simulink model "sil_test"  (R2022b)
settings: Solver=VariableStepAuto  StartTime=0.0  StopTime=inf  RelTol=1e-3
undefined symbols (not defined in the file): battery_monitor, battery_monitor_lib, BM_STATUSES, canChannel, DI_STATUSES, driver_interface, driver_interface_lib, Ended, governor, governor_lib, MI_STATUSES, motor_interface, motor_interface_lib, simp_vd_interface, simp_vd_lib, Single
libraries: canmsglib x16, canlib x10, simulink x6, speedgoatlib_IO191 x5, slrealtimeiplib x3, AMK_comms_plant_lib x1, BMS_plant_lib x1, speedgoatlib_IO614 x1, slrealtimeutilitieslib x1, etargetslib x1
(part 1 of 3)
settings Model: Creator=maxfa  LastModifiedBy=maxfa

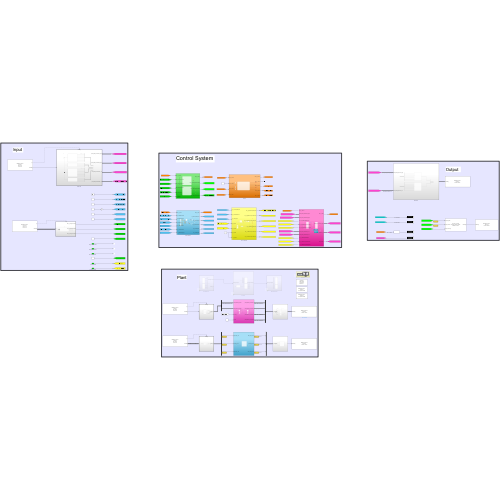
[thumbnail: Simulink's stored preview of the top-level diagram]
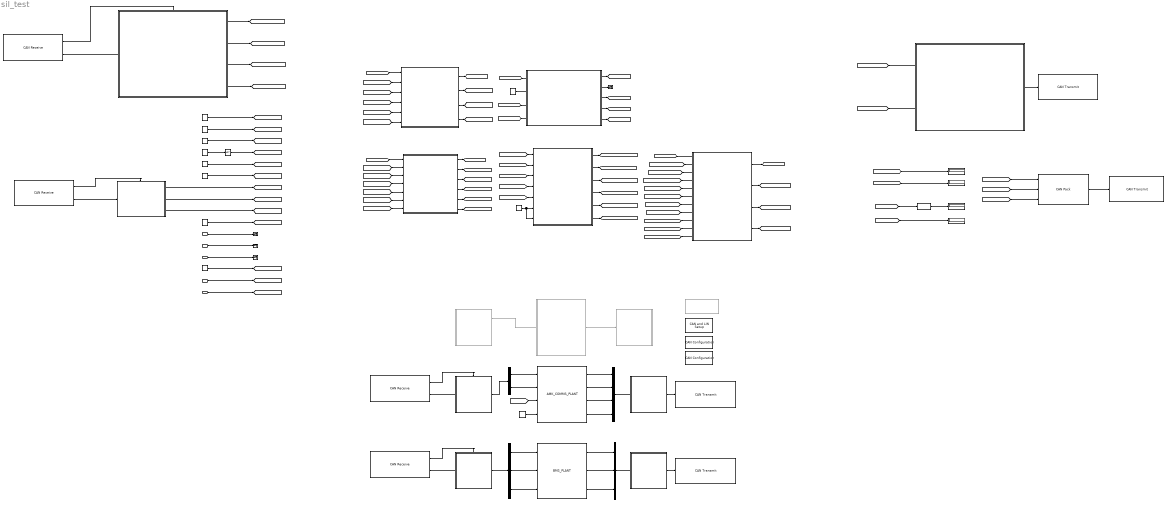
== system sil_test ==
  note: Plant
  note: Control System
  note: Input
  note: Output
  BM_LowThermValue : Inport  OutDataTypeStr=int8  Unit=°C
  BM_HighThermValue : Inport  Port=2  OutDataTypeStr=int8  Unit=°C
  BM_AvgThermValue : Inport  Port=3  OutDataTypeStr=int8  Unit=°C
  VD_LFWheelSpeed : Inport  Port=4  OutDataTypeStr=int16  Unit=rpm
  VD_RFWheelSpeed : Inport  Port=5  OutDataTypeStr=int16  Unit=rpm
  AMK_COMMS_PLANT : AMK_comms_plant_lib/AMK_COMMS_PLANT  SystemSampleTime=-1  VariantActivationTime=update diagram  Latency=0  AutoFrameSizeCalculation=off
  AMK_Input : Subsystem  TreatAsAtomicUnit=on
  AMK_Output : Subsystem
  BMS_PLANT : BMS_plant_lib/BMS_PLANT  SystemSampleTime=-1  VariantActivationTime=update diagram  Latency=0  AutoFrameSizeCalculation=off
  Bus Creator : BusCreator  Inputs=4
  Bus Creator1 : BusCreator  Inputs=3
  Bus Selector : BusSelector  OutputSignals=ptCAN_AMK0_Setpoints1_Left,ptCAN_AMK1_Setpoints1_Right
  Bus Selector1 : BusSelector  OutputSignals=AIR_pos,precharge,AIR_neg
  CAN Configuration : canlib/CAN Configuration  BlockHandle=2172.0005  Device=MathWorks Virtual 1 (Channel 1)  DeviceMenu=MathWorks Virtual 1 (Channel 1)  ObjConstructor=canChannel('MathWorks', 'Virtual 1', 1)  BusSpeed=500000  EnableBitParameters=off  AckMode=Normal
  CAN Configuration1 : canlib/CAN Configuration  BlockHandle=2172.0005  Device=MathWorks Virtual 1 (Channel 2)  DeviceMenu=MathWorks Virtual 1 (Channel 2)  ObjConstructor=canChannel('MathWorks', 'Virtual 1', 2)  BusSpeed=500000  EnableBitParameters=off  AckMode=Normal
  CAN Pack : canmsglib/CAN Pack  CANdbFile=C:\Users\maxfa\Documents\vehicle_control_system\src\testing\Vehicle_HIL_plant\VEH_CAN.dbc  MsgList=Contactor_States  MsgName=Contactor_States  MsgIDType=Standard (11-bit identifier)  MsgIdentifier=1570  MsgLength=3  Remote=off  ApplyMinMax=off  BusOutput=off  SignalInfo={'Pack_Negative','16','8','LE','unsigned','Standard','0','1','0','-Inf','Inf';'Pack_Positive','0','8','LE','unsigned','Standard','0','1','0','-Inf','Inf';'Pack_Precharge','8','8','LE','unsigned','Standard','0','1','0','-Inf','Inf'}
      settings: LibrarySourceBlock=canlib/CAN Pack  DataFormat=CANdb specified signals
  CAN Receive : canlib/CAN Receive  BlockHandle=204.0002  Device=MathWorks Virtual 1 (Channel 1)  DeviceMenu=MathWorks Virtual 1 (Channel 1)  ObjConstructor=canChannel('MathWorks', 'Virtual 1', 1)  EnableStandardIDsFilter=off  StdIDsCombo=Allow all  StandardIDs=0  EnableExtendedIDsFilter=off  ExtIDsCombo=Allow all  ExtendedIDs=0  SampleTime=0.005  MsgsPerTimestep=all  InternalFilterUpdateStatus=on  BusOutput=off
  CAN Receive1 : canlib/CAN Receive  BlockHandle=207.0002  Device=MathWorks Virtual 1 (Channel 1)  DeviceMenu=MathWorks Virtual 1 (Channel 1)  ObjConstructor=canChannel('MathWorks', 'Virtual 1', 1)  EnableStandardIDsFilter=off  StdIDsCombo=Allow all  StandardIDs=0  EnableExtendedIDsFilter=off  ExtIDsCombo=Allow all  ExtendedIDs=0  SampleTime=0.005  MsgsPerTimestep=all  InternalFilterUpdateStatus=on  BusOutput=off
  CAN Receive2 : canlib/CAN Receive  BlockHandle=210.0002  Device=MathWorks Virtual 1 (Channel 2)  DeviceMenu=MathWorks Virtual 1 (Channel 2)  ObjConstructor=canChannel('MathWorks', 'Virtual 1', 2)  EnableStandardIDsFilter=off  StdIDsCombo=Allow all  StandardIDs=0  EnableExtendedIDsFilter=off  ExtIDsCombo=Allow all  ExtendedIDs=0  SampleTime=0.005  MsgsPerTimestep=all  InternalFilterUpdateStatus=on  BusOutput=on
  CAN Receive4 : canlib/CAN Receive  BlockHandle=213.0002  Device=MathWorks Virtual 1 (Channel 2)  DeviceMenu=MathWorks Virtual 1 (Channel 2)  ObjConstructor=canChannel('MathWorks', 'Virtual 1', 2)  EnableStandardIDsFilter=off  StdIDsCombo=Allow all  StandardIDs=0  EnableExtendedIDsFilter=off  ExtIDsCombo=Allow all  ExtendedIDs=0  SampleTime=0.005  MsgsPerTimestep=all  InternalFilterUpdateStatus=on  BusOutput=on
  CAN Transmit : canlib/CAN Transmit  BlockHandle=216.0002  Device=MathWorks Virtual 1 (Channel 1)  DeviceMenu=MathWorks Virtual 1 (Channel 1)  ObjConstructor=canChannel('MathWorks', 'Virtual 1', 1)  EnableEventTransmit=off  EnablePeriodicTransmit=on  MessagePeriod=0.005
  CAN Transmit1 : canlib/CAN Transmit  BlockHandle=218.0002  Device=MathWorks Virtual 1 (Channel 1)  DeviceMenu=MathWorks Virtual 1 (Channel 1)  ObjConstructor=canChannel('MathWorks', 'Virtual 1', 1)  EnableEventTransmit=off  EnablePeriodicTransmit=on  MessagePeriod=0.005
  CAN Transmit2 : canlib/CAN Transmit  BlockHandle=3044.0012  Device=MathWorks Virtual 1 (Channel 2)  DeviceMenu=MathWorks Virtual 1 (Channel 2)  ObjConstructor=canChannel('MathWorks', 'Virtual 1', 2)  EnableEventTransmit=off  EnablePeriodicTransmit=on  MessagePeriod=0.005
  CAN Transmit4 : canlib/CAN Transmit  BlockHandle=220.0002  Device=MathWorks Virtual 1 (Channel 2)  DeviceMenu=MathWorks Virtual 1 (Channel 2)  ObjConstructor=canChannel('MathWorks', 'Virtual 1', 2)  EnableEventTransmit=off  EnablePeriodicTransmit=on  MessagePeriod=0.005
  "CAN and LIN Setup " : speedgoatlib_IO614/CAN and LIN Setup   moduleInitValues="[614    1    1   -1   -1]"  id=1  moduleType=IO614  pciSlot=-1  canChn1=CAN (HS)  canChn2=CAN (HS)  canChn3=Disabled  canChn4=Disabled  linChn1=Disabled  linChn2=Disabled  canInitStructArray=[]  canTermStructArray=[]  canChn1InitValues="[2   4   1  31   8   2   1   5   2]"  arbBdrChn1=500 kBaud  arbManBdrChn1=[4,1,31,8]  fdBdrChn1=5.0 MBaud  fdManBdrChn1=[2,1,5,2]  canChn2InitValues="[2   4   1  31   8   2   1   5   2]"  arbBdrChn2=500 kBaud  arbManBdrChn2=[4,1,31,8]  fdBdrChn2=5.0 MBaud  fdManBdrChn2=[2,1,5,2]  canChn3InitValues="[1   2   1  31   8   2   1   5   2]"  arbBdrChn3=1.0 MBaud  arbManBdrChn3=[2,1,31,8]  fdBdrChn3=5.0 MBaud  fdManBdrChn3=[2,1,5,2]  canChn4InitValues="[1   2   1  31   8   2   1   5   2]"  arbBdrChn4=1.0 MBaud  arbManBdrChn4=[2,1,31,8]  fdBdrChn4=5.0 MBaud  fdManBdrChn4=[2,1,5,2]  bdrLIN1=19200  linChn1InitValues="[1  19200]"  bdrLIN2=19200  linChn2InitValues="[1  19200]"
      settings: LibrarySourceBlock=speedgoatlib_CANLIN_OfA2/CAN and LIN Setup
  Cast To Single : DataTypeConversion  OutDataTypeStr=uint8  SaturateOnIntegerOverflow=off  RndMeth=Floor
  Constant : Constant  Value=0
  Constant1 : Constant  Value=0
  Constant13 : Constant  Value=0  OutMin=0  OutMax=1
  Constant14 : Constant  Value=100  OutMin=0  OutMax=100
  Constant2 : Constant  Value=0
  Constant4 : Constant  Value=0.5066380718954249  OutMin=0  OutMax=1
  Constant5 : Constant  OutMin=0  OutMax=1
  Constant6 : Constant  OutMin=0  OutMax=1
  Constant7 : Constant  Value=0  OutMin=0  OutMax=1
  Constant8 : Constant  Value=0  OutMin=0  OutMax=1
  Constant9 : Constant  Value=0.02343014359698682  OutMin=0  OutMax=1
  Dashboard : Subsystem  Commented=on
  Display{,1..3} (4 alike) : Display
  Function-Call Subsystem : Subsystem  TreatAsAtomicUnit=on
  Function-Call Subsystem1 : Subsystem  TreatAsAtomicUnit=on
  Function-Call Subsystem2 : Subsystem  TreatAsAtomicUnit=on
  NOT : Logic  Operator=NOT  IconShape=distinctive  AllPortsSameDT=off  OutDataTypeStr=boolean
  Speedgoat Inputs : Subsystem  Commented=on
  Speedgoat Outputs : Subsystem  Commented=on
  Subsystem : Subsystem
  Subsystem1 : Subsystem
  TCP Server : Subsystem  Commented=on
  Terminator{,1..3} (4 alike) : Terminator
  battery_monitor : Subsystem  AncestorBlock=battery_monitor_lib/battery_monitor
  driver_interface : Subsystem  AncestorBlock=driver_interface_lib/driver_interface
  governor : Subsystem  AncestorBlock=governor_lib/governor
  motor_interface : Subsystem  AncestorBlock=motor_interface_lib/motor_interface
  simp_vd_interface : Subsystem  AncestorBlock=simp_vd_lib/simp_vd_interface
  wires:
  Function-Call Subsystem1/1(pt_CAN_IN) -> Bus Selector1/1
  Bus Selector1/2 -> BMS_PLANT/2  "<precharge>"
  BMS_PLANT/3 -> Bus Creator1/3  "AIR_neg_sts"
  Subsystem1/1(Out1) -> CAN Transmit4/1
  Bus Selector1/1 -> BMS_PLANT/1  "<AIR_pos>"
  AMK_COMMS_PLANT/4 -> Bus Creator/4  "ptCAN_AMK1_ActualValues2"
  CAN Receive2/2 -> Function-Call Subsystem1/1(In1)
  BMS_PLANT/2 -> Bus Creator1/2  "precharge_sts"
  AMK_COMMS_PLANT/3 -> Bus Creator/3  "ptCAN_AMK1_ActualValues1"
  Subsystem/1(Out1) -> CAN Transmit1/1
  TCP Server/1(Speedgoat Outputs) -> Speedgoat Outputs/1(Speedgoat Outputs)
  AMK_COMMS_PLANT/2 -> Bus Creator/2  "ptCAN_AMK0_ActualValues2"
  Bus Creator1/1 -> Subsystem1/1(pt_CAN_OUT)
  CAN Receive1/2 -> Function-Call Subsystem/1(In1)
  Function-Call Subsystem/1(pt_CAN_IN) -> Bus Selector/1
  Constant/1 -> AMK_COMMS_PLANT/4
  Bus Selector1/3 -> BMS_PLANT/3  "<AIR_neg>"
  BMS_PLANT/1 -> Bus Creator1/1  "AIR_pos_sts"
  Bus Creator/1 -> Subsystem/1(pt_CAN_OUT)
  Bus Selector/2 -> AMK_COMMS_PLANT/2  "<ptCAN_AMK1_Setpoints1_Right>"
  AMK_COMMS_PLANT/1 -> Bus Creator/1  "ptCAN_AMK0_ActualValues1"
  Bus Selector/1 -> AMK_COMMS_PLANT/1  "<ptCAN_AMK0_Setpoints1_Left>"
  Speedgoat Inputs/1(Speedgoat Inputs) -> TCP Server/1(Speedgoat Inputs)
  [BM_b_prechargeContactorCMD] -> CAN Pack/3
  BM_AvgThermValue/1 -> Terminator3/1
  motor_interface/2(ptCAN_AMK_Setpoints1_Right) -> [ptCAN_AMK_Setpoints1_Right]
  Constant14/1 -> [BM_PackSOC]
  BM_HighThermValue/1 -> Terminator2/1
  [BM_PackSOC] -> battery_monitor/6(BM_PackSOC)
  VD_LFWheelSpeed/1 -> [VD_LFWheelSpeed]
  Constant6/1 -> [DI_RearBrakePressure]
  [BM_HVnegContactorSts] -> battery_monitor/4(BM_HVnegContactorSts)
  [VD_RFWheelSpeed] -> simp_vd_interface/5(DI_p_wspdRF)
  battery_monitor/4(BM_b_HVnegContactorCMD) -> [BM_b_HVnegContactorCMD]
  [VD_LFWheelSpeed] -> simp_vd_interface/4(DI_p_wspdLF)
  VD_RFWheelSpeed/1 -> [VD_RFWheelSpeed]
  Constant4/1 -> [DI_SteeringAngle]
  [DI_StartButton] -> driver_interface/4(DI_StartButton)
  motor_interface/1(GOV_e_miSts) -> [GOV_e_miSts]
  BM_LowThermValue/1 -> Terminator1/1
  [GOV_e_miCmd] -> motor_interface/1(GOV_e_miCmd)
  [BM_HvilFeedback] -> battery_monitor/5(BM_HvilFeedback)
  [DI_AccelPedalPosition2] -> driver_interface/6(DI_V_AccelPedalPos2)
  [DI_b_brakeLightEn] -> Display1/1  "DI_b_brakeLightEn"
  [GOV_e_diSts] -> governor/4(GOV_e_diSts)
  Cast To Single/1 -> Display2/1
  [DI_p_brakePedalPosition] -> simp_vd_interface/2(DI_p_brakePedalPosition)
  [GOV_e_govSts] -> Cast To Single/1  "GOV_e_govSts"
  [MI_InverterEn] -> Display3/1
  simp_vd_interface/1(VD_n_RightMotorSpeedRequest) -> [VD_n_RightMotorSpeedRequest]
  governor/4(GOV_e_diCmd) -> [GOV_e_diCmd]
  [DI_RearBrakePressure] -> driver_interface/3(DI_RearBrakePressure)
  motor_interface/4(MI_InverterEn) -> [MI_InverterEn]
  battery_monitor/2(BM_b_prechargeContactorCMD) -> [BM_b_prechargeContactorCMD]
  [GOV_e_diCmd] -> driver_interface/1(GOV_e_diCmd)
  [DI_AccelPedalPosition1] -> driver_interface/5(DI_V_AccelPedalPos1)
  [ptCAN_AMK_ActualValues2_Left] -> motor_interface/8(ptCAN_AMK_ActualValues2_Left)
  [DI_SteeringAngle] -> driver_interface/7(Dl_V_RawSteeringAngle)
  simp_vd_interface/3(VD_T_RightMotorTorqueLimitNegative) -> [VD_T_RightMotorTorqueLimitNegative]
  [DI_FrontBrakePressure] -> driver_interface/2(DI_FrontBrakePressure)
  governor/5(GOV_e_govSts) -> [GOV_e_govSts]
  [BM_prechrgContactorSts] -> battery_monitor/2(BM_prechrgContactorSts)
  driver_interface/6(DI_b_brakeLightEn) -> [DI_b_brakeLightEn]
  simp_vd_interface/6(VD_T_LeftMotorTorqueLimitNegative) -> [VD_T_LeftMotorTorqueLimitNegative]
  simp_vd_interface/5(VD_T_LeftMotorTorqueLimitPositive) -> [VD_T_LeftMotorTorqueLimitPositive]
  [ptCAN_AMK_ActualValues1_Left] -> motor_interface/7(ptCAN_AMK_ActualValues1_Left)
  simp_vd_interface/2(VD_T_RightMotorTorqueLimitPositive) -> [VD_T_RightMotorTorqueLimitPositive]
  Constant13/1 -> [BM_HvilFeedback]
  [DI_p_driverTorqueRequest] -> simp_vd_interface/1(DI_p_driverTorqueRequest)
  [GOV_e_bmCmd] -> battery_monitor/1(GOV_e_bmCmd)
  simp_vd_interface/4(VD_n_LeftMotorSpeedRequest) -> [VD_n_LeftMotorSpeedRequest]
  Constant5/1 -> [DI_FrontBrakePressure]
  [VD_T_LeftMotorTorqueLimitPositive] -> motor_interface/10(VD_T_LeftMotorTorqueLimitPositive)
  [ptCAN_AMK_ActualValues2_Right] -> motor_interface/3(ptCAN_AMK_ActualValues2_Right)
  Function-Call Subsystem2/1(BM_b_prechrgContactorSts) -> [BM_prechrgContactorSts]
  governor/1(GOV_e_bmCmd) -> [GOV_e_bmCmd]
  [GOV_e_miSts] -> governor/3(GOV_e_miSts)
  governor/3(GOV_e_miCmd) -> [GOV_e_miCmd]
  Function-Call Subsystem2/3(BM_b_HVnegContactorSts) -> [BM_HVnegContactorSts]
  Constant9/1 -> [DI_AccelPedalPosition2]
  [BM_HVposContactorSts] -> battery_monitor/3(BM_HVposContactorSts)
  [VD_n_RightMotorSpeedRequest] -> motor_interface/4(VD_n_RightMotorSpeedRequest)
  [VD_T_RightMotorTorqueLimitNegative] -> motor_interface/6(VD_T_RightMotorTorqueLimitNegative)
  driver_interface/2(DI_driverTorqueRequest) -> [DI_p_driverTorqueRequest]
  Constant7/1 -> NOT/1
  Constant1/1 -> governor/2(GOV_e_vdSts)
  driver_interface/1(GOV_e_diSts) -> [GOV_e_diSts]
  [GOV_e_bmSts] -> governor/1(GOV_e_bmSts)
  [VD_T_RightMotorTorqueLimitPositive] -> motor_interface/5(VD_T_RightMotorTorqueLimitPositive)
  Function-Call Subsystem2/2(BM_b_HVposContactorSts) -> [BM_HVposContactorSts]
  driver_interface/5(DI_b_driverSpeaker) -> [DI_b_driverSpeaker]
  driver_interface/3(DI_p_steeringAngle) -> [DI_p_steeringAngle]
  driver_interface/4(DI_p_brakePedalPos) -> [DI_p_brakePedalPosition]
  [ptCAN_AMK_ActualValues1_Right] -> motor_interface/2(ptCAN_AMK_ActualValues1_Right)
  [VD_T_LeftMotorTorqueLimitNegative] -> motor_interface/11(VD_T_LeftMotorTorqueLimitNegative)
  [DI_p_steeringAngle] -> simp_vd_interface/3(DI_p_steeringAngle)
  Constant8/1 -> [DI_AccelPedalPosition1]
  [DI_b_driverSpeaker] -> Display/1  "DI_b_driverSpeaker"
  governor/2(GOV_e_vdCmd) -> Terminator/1
  battery_monitor/1(GOV_e_bmSts) -> [GOV_e_bmSts]
  motor_interface/3(ptCAN_AMK_Setpoints1_Left) -> [ptCAN_AMK_Setpoints1_Left]
  [VD_n_LeftMotorSpeedRequest] -> motor_interface/9(VD_n_LeftMotorSpeedRequest)
  battery_monitor/3(BM_b_HVposContactorCMD) -> [BM_b_HVposContactorCMD]
  Constant2/1 -> simp_vd_interface/7(DI_p_wspdLRR), simp_vd_interface/6(DI_p_wspdLR)
  CAN Receive/1 -> AMK_Input/Trigger
  AMK_Input/4(ptCAN_AMK_ActualValues2_Left) -> [ptCAN_AMK_ActualValues2_Left]
  AMK_Input/2(ptCAN_AMK_ActualValues2_Right) -> [ptCAN_AMK_ActualValues2_Right]
  CAN Receive/2 -> AMK_Input/1(In1)
  AMK_Input/1(ptCAN_AMK_ActualValues1_Right) -> [ptCAN_AMK_ActualValues1_Right]
  AMK_Input/3(ptCAN_AMK_ActualValues1_Left) -> [ptCAN_AMK_ActualValues1_Left]
  CAN Receive4/2 -> Function-Call Subsystem2/1(In1)
  CAN Receive4/1 -> Function-Call Subsystem2/Trigger
  AMK_Output/1(Out1) -> CAN Transmit/1
  [ptCAN_AMK_Setpoints1_Right] -> AMK_Output/1(ptCAN_AMK_Setpoints1_Right)  "ptCAN_AMK_Setpoints1_Right"
  [ptCAN_AMK_Setpoints1_Left] -> AMK_Output/2(ptCAN_AMK_Setpoints1_Left)  "ptCAN_AMK_Setpoints1_Left"
  CAN Receive1/1 -> Function-Call Subsystem/Trigger
  CAN Receive2/1 -> Function-Call Subsystem1/Trigger
  [MI_InverterEn] -> AMK_COMMS_PLANT/3
  NOT/1 -> [DI_StartButton]
  CAN Pack/1 -> CAN Transmit2/1
  [BM_b_HVposContactorCMD] -> CAN Pack/2
  [BM_b_HVnegContactorCMD] -> CAN Pack/1

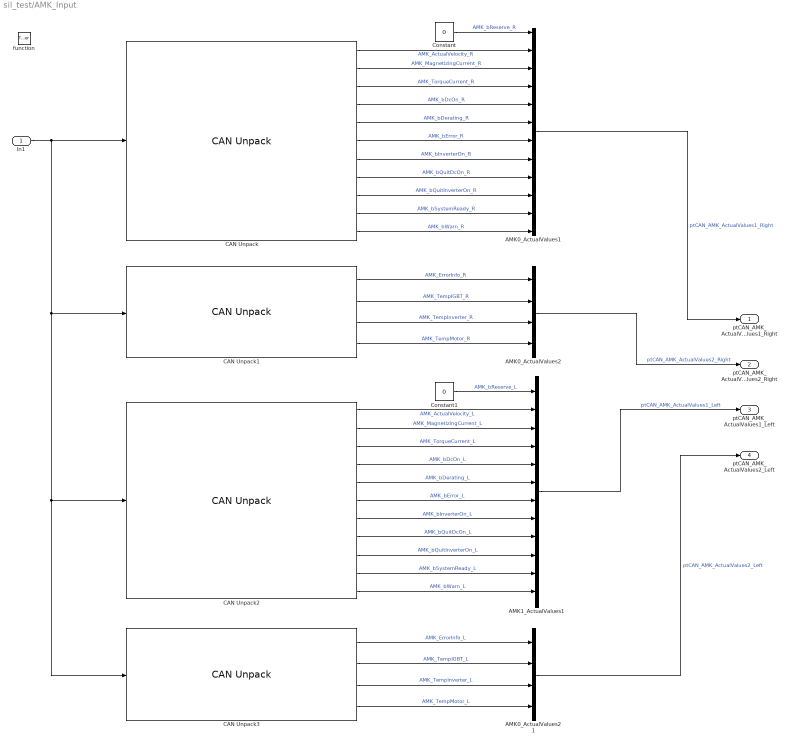
== system sil_test/AMK_Input ==
  In1 : Inport
  function : TriggerPort  TriggerType=function-call  VariantControl=(inherit)
  "AMK0_ActualValues1 " : BusCreator  Inputs=12
  "AMK0_ActualValues2 " : BusCreator  Inputs=4
  AMK0_ActualValues2 1 : BusCreator  Inputs=4
  AMK1_ActualValues1 : BusCreator  Inputs=12
  CAN Unpack : canmsglib/CAN Unpack  CANdbFile=C:\Users\maxfa\OneDrive\Documents\vehicle_control_system\src\testing\Plant\Bench\CAN_Databases-master\CAN_AMKInverter.dbc  MsgList=AMK1_ActualValues1  MsgName=AMK1_ActualValues1  MsgIDType=Standard (11-bit identifier)  MsgIdentifier=645  MsgLength=8  SignalInfo={'AMK_ActualVelocity','16','16','LE','signed','Standard','0','1','0','-Inf','Inf';'AMK_MagnetizingCurrent','48','16','LE','signed','Standard','0','1','0','-Inf','Inf';'AMK_TorqueCurrent','32','16','LE','signed','Standard','0','1','0','-Inf','Inf';'AMK_bDcOn','12','1','LE','unsigned','Standard','0','1','0','-Inf','Inf';'AMK_bDerating','15','1','LE','unsigned','Standard','0','1','0','-Inf','Inf';'AMK_bError','9','1','LE','unsigned','Standard','0','1','0','-Inf','Inf';'AMK_bInverterOn','14','1','LE','unsigned','Standard','0','1','0','-Inf','Inf';'AMK_bQuitDcOn','11','1','LE','unsigned','Standard','0','1','0','-Inf','Inf';'AMK_bQuitInverterOn','13','1','LE','unsigned','Standard','0','1','0','-Inf','Inf';'AMK_bSystemReady','8','1','LE','unsigned','Standard','0','1','0','-Inf','Inf';'AMK_bWarn','10','1','LE','unsigned','Standard','0','1','0','-Inf','Inf'}  IDPort=off  TimestampPort=off  ErrorPort=off  RemotePort=off  LengthPort=off  StatusPort=off  ApplyMinMax=off
      settings: LibrarySourceBlock=canlib/CAN Unpack  DataFormat=CANdb specified signals
  CAN Unpack1 : canmsglib/CAN Unpack  CANdbFile=C:\Users\maxfa\OneDrive\Documents\vehicle_control_system\src\testing\Plant\Bench\CAN_Databases-master\CAN_AMKInverter.dbc  MsgList=AMK1_ActualValues2  MsgName=AMK1_ActualValues2  MsgIDType=Standard (11-bit identifier)  MsgIdentifier=647  MsgLength=8  SignalInfo={'AMK_ErrorInfo','32','16','LE','unsigned','Standard','0','1','0','0','65535';'AMK_TempIGBT','48','16','LE','signed','Standard','0','0.1','0','-3276.8','3276.7';'AMK_TempInverter','16','16','LE','signed','Standard','0','0.1','0','-3276.8','3276.7';'AMK_TempMotor','0','16','LE','signed','Standard','0','0.1','0','-3276.8','3276.7'}  IDPort=off  TimestampPort=off  ErrorPort=off  RemotePort=off  LengthPort=off  StatusPort=off  ApplyMinMax=off
      settings: LibrarySourceBlock=canlib/CAN Unpack  DataFormat=CANdb specified signals
  CAN Unpack2 : canmsglib/CAN Unpack  CANdbFile=C:\Users\maxfa\OneDrive\Documents\vehicle_control_system\src\testing\Plant\Bench\CAN_Databases-master\CAN_AMKInverter.dbc  MsgList=AMK0_ActualValues1  MsgName=AMK0_ActualValues1  MsgIDType=Standard (11-bit identifier)  MsgIdentifier=644  MsgLength=8  SignalInfo={'AMK_ActualVelocity','16','16','LE','signed','Standard','0','1','0','-Inf','Inf';'AMK_MagnetizingCurrent','48','16','LE','signed','Standard','0','1','0','-Inf','Inf';'AMK_TorqueCurrent','32','16','LE','signed','Standard','0','1','0','-Inf','Inf';'AMK_bDcOn','12','1','LE','unsigned','Standard','0','1','0','-Inf','Inf';'AMK_bDerating','15','1','LE','unsigned','Standard','0','1','0','-Inf','Inf';'AMK_bError','9','1','LE','unsigned','Standard','0','1','0','-Inf','Inf';'AMK_bInverterOn','14','1','LE','unsigned','Standard','0','1','0','-Inf','Inf';'AMK_bQuitDcOn','11','1','LE','unsigned','Standard','0','1','0','-Inf','Inf';'AMK_bQuitInverterOn','13','1','LE','unsigned','Standard','0','1','0','-Inf','Inf';'AMK_bSystemReady','8','1','LE','unsigned','Standard','0','1','0','-Inf','Inf';'AMK_bWarn','10','1','LE','unsigned','Standard','0','1','0','-Inf','Inf'}  IDPort=off  TimestampPort=off  ErrorPort=off  RemotePort=off  LengthPort=off  StatusPort=off  ApplyMinMax=off
      settings: LibrarySourceBlock=canlib/CAN Unpack  DataFormat=CANdb specified signals
  CAN Unpack3 : canmsglib/CAN Unpack  CANdbFile=C:\Users\maxfa\OneDrive\Documents\vehicle_control_system\src\testing\Plant\Bench\CAN_Databases-master\CAN_AMKInverter.dbc  MsgList=AMK0_ActualValues2  MsgName=AMK0_ActualValues2  MsgIDType=Standard (11-bit identifier)  MsgIdentifier=646  MsgLength=8  SignalInfo={'AMK_ErrorInfo','32','16','LE','unsigned','Standard','0','1','0','0','65535';'AMK_TempIGBT','48','16','LE','signed','Standard','0','0.1','0','-3276.8','3276.7';'AMK_TempInverter','16','16','LE','signed','Standard','0','0.1','0','-3276.8','3276.7';'AMK_TempMotor','0','16','LE','signed','Standard','0','0.1','0','-3276.8','3276.7'}  IDPort=off  TimestampPort=off  ErrorPort=off  RemotePort=off  LengthPort=off  StatusPort=off  ApplyMinMax=off
      settings: LibrarySourceBlock=canlib/CAN Unpack  DataFormat=CANdb specified signals
  Constant : Constant  Value=0
  Constant1 : Constant  Value=0
  ptCAN_AMK_ActualValues1_Right : Outport
  ptCAN_AMK_ActualValues2_Right : Outport  Port=2
  ptCAN_AMK_ActualValues1_Left : Outport  Port=3
  ptCAN_AMK_ActualValues2_Left : Outport  Port=4
  wires:
  In1/1 -> CAN Unpack3/1, CAN Unpack2/1, CAN Unpack1/1, CAN Unpack/1
  CAN Unpack/1 -> "AMK0_ActualValues1 "/2  "AMK_ActualVelocity_R"
  CAN Unpack/2 -> "AMK0_ActualValues1 "/3  "AMK_MagnetizingCurrent_R"
  CAN Unpack/3 -> "AMK0_ActualValues1 "/4  "AMK_TorqueCurrent_R"
  CAN Unpack/4 -> "AMK0_ActualValues1 "/5  "AMK_bDcOn_R"
  CAN Unpack/5 -> "AMK0_ActualValues1 "/6  "AMK_bDerating_R"
  CAN Unpack/6 -> "AMK0_ActualValues1 "/7  "AMK_bError_R"
  CAN Unpack/7 -> "AMK0_ActualValues1 "/8  "AMK_bInverterOn_R"
  CAN Unpack/8 -> "AMK0_ActualValues1 "/9  "AMK_bQuitDcOn_R"
  CAN Unpack/9 -> "AMK0_ActualValues1 "/10  "AMK_bQuitInverterOn_R"
  CAN Unpack/10 -> "AMK0_ActualValues1 "/11  "AMK_bSystemReady_R"
  CAN Unpack/11 -> "AMK0_ActualValues1 "/12  "AMK_bWarn_R"
  "AMK0_ActualValues1 "/1 -> ptCAN_AMK_ActualValues1_Right/1  "ptCAN_AMK_ActualValues1_Right"
  CAN Unpack2/1 -> AMK1_ActualValues1/2  "AMK_ActualVelocity_L"
  CAN Unpack2/10 -> AMK1_ActualValues1/11  "AMK_bSystemReady_L"
  CAN Unpack2/6 -> AMK1_ActualValues1/7  "AMK_bError_L"
  CAN Unpack2/9 -> AMK1_ActualValues1/10  "AMK_bQuitInverterOn_L"
  CAN Unpack2/2 -> AMK1_ActualValues1/3  "AMK_MagnetizingCurrent_L"
  CAN Unpack2/3 -> AMK1_ActualValues1/4  "AMK_TorqueCurrent_L"
  AMK1_ActualValues1/1 -> ptCAN_AMK_ActualValues1_Left/1  "ptCAN_AMK_ActualValues1_Left"
  CAN Unpack2/8 -> AMK1_ActualValues1/9  "AMK_bQuitDcOn_L"
  CAN Unpack2/4 -> AMK1_ActualValues1/5  "AMK_bDcOn_L"
  CAN Unpack2/5 -> AMK1_ActualValues1/6  "AMK_bDerating_L"
  CAN Unpack2/11 -> AMK1_ActualValues1/12  "AMK_bWarn_L"
  CAN Unpack2/7 -> AMK1_ActualValues1/8  "AMK_bInverterOn_L"
  CAN Unpack1/1 -> "AMK0_ActualValues2 "/1  "AMK_ErrorInfo_R"
  CAN Unpack1/2 -> "AMK0_ActualValues2 "/2  "AMK_TempIGBT_R"
  CAN Unpack1/3 -> "AMK0_ActualValues2 "/3  "AMK_TempInverter_R"
  CAN Unpack1/4 -> "AMK0_ActualValues2 "/4  "AMK_TempMotor_R"
  "AMK0_ActualValues2 "/1 -> ptCAN_AMK_ActualValues2_Right/1  "ptCAN_AMK_ActualValues2_Right"
  CAN Unpack3/1 -> AMK0_ActualValues2 1/1  "AMK_ErrorInfo_L"
  CAN Unpack3/4 -> AMK0_ActualValues2 1/4  "AMK_TempMotor_L"
  AMK0_ActualValues2 1/1 -> ptCAN_AMK_ActualValues2_Left/1  "ptCAN_AMK_ActualValues2_Left"
  CAN Unpack3/3 -> AMK0_ActualValues2 1/3  "AMK_TempInverter_L"
  CAN Unpack3/2 -> AMK0_ActualValues2 1/2  "AMK_TempIGBT_L"
  Constant/1 -> "AMK0_ActualValues1 "/1  "AMK_bReserve_R"
  Constant1/1 -> AMK1_ActualValues1/1  "AMK_bReserve_L"

== system sil_test/AMK_Output ==
  ptCAN_AMK_Setpoints1_Right : Inport
  ptCAN_AMK_Setpoints1_Left : Inport  Port=2
  Bus Creator : BusCreator  Inputs=2
  Bus Selector : BusSelector  OutputSignals=AMK_TargetVelocity,AMK_TorqueLimitNegativ,AMK_TorqueLimitPositiv,AMK_bDcOn,AMK_bEnable,AMK_bErrorReset,AMK_bInverterOn
  Bus Selector1 : BusSelector  OutputSignals=AMK_TargetVelocity,AMK_TorqueLimitNegativ,AMK_TorqueLimitPositiv,AMK_bDcOn,AMK_bEnable,AMK_bErrorReset,AMK_bInverterOn
  CAN Pack : canmsglib/CAN Pack  CANdbFile=C:\Users\maxfa\OneDrive\Documents\vehicle_control_system\src\testing\Plant\Bench\CAN_Databases-master\CAN_AMKInverter.dbc  MsgList=AMK1_SetPoints1  MsgName=AMK1_SetPoints1  MsgIDType=Standard (11-bit identifier)  MsgIdentifier=390  MsgLength=8  Remote=off  ApplyMinMax=off  BusOutput=off  SignalInfo={'AMK_TargetVelocity','16','16','LE','signed','Standard','0','1','0','-Inf','Inf';'AMK_TorqueLimitNegativ','48','16','LE','signed','Standard','0','1','0','-Inf','Inf';'AMK_TorqueLimitPositiv','32','16','LE','signed','Standard','0','1','0','-Inf','Inf';'AMK_bDcOn','9','1','LE','unsigned','Standard','0','1','0','-Inf','Inf';'AMK_bEnable','10','1','LE','unsigned','Standard','0','1','0','-Inf','Inf';'AMK_bErrorReset','11','1','LE','unsigned','Standard','0','1','0','-Inf','Inf';'AMK_bInverterOn','8','1','LE','unsigned','Standard','0','1','0','-Inf','Inf'}
      settings: LibrarySourceBlock=canlib/CAN Pack  DataFormat=CANdb specified signals
  CAN Pack1 : canmsglib/CAN Pack  CANdbFile=C:\Users\maxfa\OneDrive\Documents\vehicle_control_system\src\testing\Plant\Bench\CAN_Databases-master\CAN_AMKInverter.dbc  MsgList=AMK0_SetPoints1  MsgName=AMK0_SetPoints1  MsgIDType=Standard (11-bit identifier)  MsgIdentifier=389  MsgLength=8  Remote=off  ApplyMinMax=off  BusOutput=off  SignalInfo={'AMK_TargetVelocity','16','16','LE','signed','Standard','0','1','0','-Inf','Inf';'AMK_TorqueLimitNegativ','48','16','LE','signed','Standard','0','1','0','-Inf','Inf';'AMK_TorqueLimitPositiv','32','16','LE','signed','Standard','0','1','0','-Inf','Inf';'AMK_bDcOn','9','1','LE','unsigned','Standard','0','1','0','-Inf','Inf';'AMK_bEnable','10','1','LE','unsigned','Standard','0','1','0','-Inf','Inf';'AMK_bErrorReset','11','1','LE','unsigned','Standard','0','1','0','-Inf','Inf';'AMK_bInverterOn','8','1','LE','unsigned','Standard','0','1','0','-Inf','Inf'}
      settings: LibrarySourceBlock=canlib/CAN Pack  DataFormat=CANdb specified signals
  Out1 : Outport
  wires:
  CAN Pack/1 -> Bus Creator/1  "AMK0_SetPoints1"
  CAN Pack1/1 -> Bus Creator/2  "AMK1_SetPoints1"
  Bus Selector/7 -> CAN Pack/7  "<AMK_bInverterOn>"
  Bus Selector/4 -> CAN Pack/4  "<AMK_bDcOn>"
  Bus Selector/5 -> CAN Pack/5  "<AMK_bEnable>"
  Bus Selector/6 -> CAN Pack/6  "<AMK_bErrorReset>"
  Bus Selector/1 -> CAN Pack/1  "<AMK_TargetVelocity>"
  Bus Selector/3 -> CAN Pack/3  "<AMK_TorqueLimitPositiv>"
  Bus Selector/2 -> CAN Pack/2  "<AMK_TorqueLimitNegativ>"
  Bus Creator/1 -> Out1/1
  Bus Selector1/1 -> CAN Pack1/1  "<AMK_TargetVelocity>"
  Bus Selector1/3 -> CAN Pack1/3  "<AMK_TorqueLimitPositiv>"
  Bus Selector1/2 -> CAN Pack1/2  "<AMK_TorqueLimitNegativ>"
  Bus Selector1/4 -> CAN Pack1/4  "<AMK_bDcOn>"
  Bus Selector1/5 -> CAN Pack1/5  "<AMK_bEnable>"
  Bus Selector1/6 -> CAN Pack1/6  "<AMK_bErrorReset>"
  Bus Selector1/7 -> CAN Pack1/7  "<AMK_bInverterOn>"
  ptCAN_AMK_Setpoints1_Right/1 -> Bus Selector/1
  ptCAN_AMK_Setpoints1_Left/1 -> Bus Selector1/1

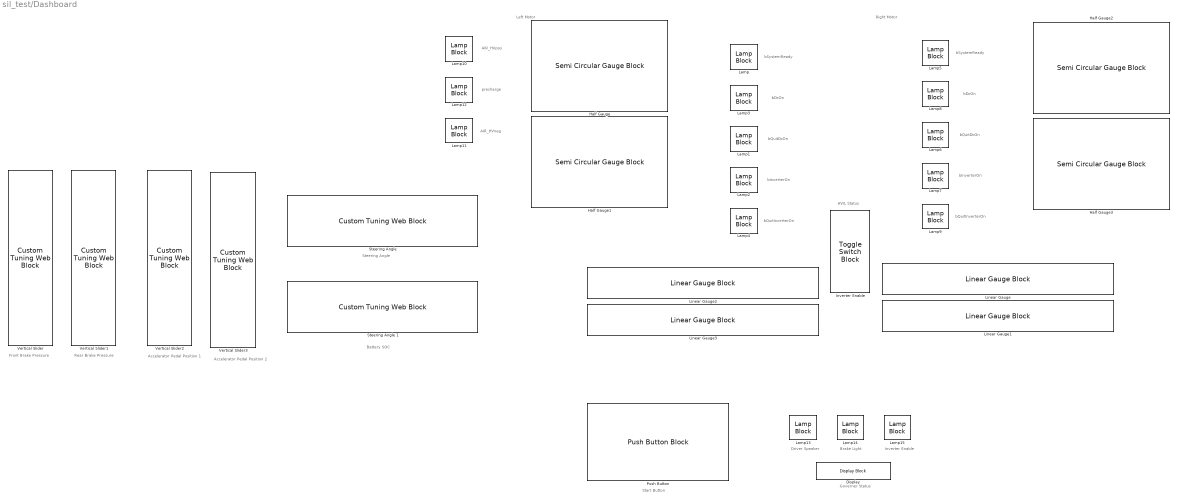
== system sil_test/Dashboard ==
  note: Front Brake Pressure
  note: HVIL Status
  note: Left Motor
  note: bQuitInverterOn
  note: bInverterOn
  note: bQuitDcOn
  note: bDcOn
  note: bSystemReady
  note: bDcOn
  note: bQuitDcOn
  note: bSystemReady
  note: bInverterOn
  note: bQuitInverterOn
  note: Right Motor
  note: AIR_HVpos
  note: precharge
  note: AIR_HVneg
  note: Rear Brake Pressure
  note: Steering Angle
  note: Start Button
  note: Accelerator Pedal
      | Position 2
  note: Accelerator Pedal Position 1
  note: Battery SOC
  note: Driver Speaker
  note: Brake Light
  note: Inverter Enable
  note: Governer Status
  Display : DisplayBlock  LabelPosition=Hide  Transparency=1
  Half Gauge : SemiCircularGaugeBlock  LabelPosition=Bottom  ScaleMax=20000  TickInterval=2000
  Half Gauge1 : SemiCircularGaugeBlock  LabelPosition=Bottom  ScaleMax=1000  TickInterval=100
  Half Gauge2 : SemiCircularGaugeBlock  LabelPosition=Bottom  ScaleMax=20000  TickInterval=2000
  Half Gauge3 : SemiCircularGaugeBlock  LabelPosition=Bottom  ScaleMax=1000  TickInterval=100
  Inverter Enable : ToggleSwitchBlock  LabelPosition=Bottom
      settings: Values={{'Off', 'On'}, [0 1]}
  Lamp{,1..15} (16 alike) : LampBlock  LabelPosition=Hide
  Linear Gauge : LinearGaugeBlock  ScaleMax=20000  TickInterval=2000
  Linear Gauge1 : LinearGaugeBlock  ScaleMax=1000  TickInterval=100
  Linear Gauge2 : LinearGaugeBlock  ScaleMax=20000  TickInterval=2000
  Linear Gauge3 : LinearGaugeBlock  ScaleMax=1000  TickInterval=100
  Push Button : PushButtonBlock  OffValue=0.000000
  "Steering Angle " : CustomTuningWebBlock  LabelPosition=Hide  ShowInitialText=on  Configuration="{\"components\":[{\"name\":\"LinearScaleComponent\",\"settings\":{\"bounds\":{\"max\":1,\"min\":0,\"tickInterval\":\"auto\"},\"internalTickHeightScaleFactor\":0.5,\"labelColor\":[255,255,200],\"labelFont\":{\"font\":\"Arial\",\"fontSize\":12},\"labelOffset\":0.05,\"labelTransparency\":1,\"needleImage\":{\"size\":[596,842],\"src\":\"data:image\\/svg+xml;base64,PD94bWwgdmVyc2lvbj0iMS4wIiBlbmNvZGluZz0idXRmLTgiPz4NCjwhLS0gR2VuZXJhdG9yOiBBZG9iZSBJbGx1c3RyYXRvciAyNS4wLjAsIFNWRyBFeHBvcnQgUGx1Zy1JbiAuIFNWRyBWZXJzaW9uOiA2LjAwIEJ1aWxkIDApICAtLT4NCjxzdmcgdmVyc2lvbj0iMS4xIg0KCSBpZD0ic3ZnOCIgeG1sbnM6Y2M9Imh0dHA6Ly9jcmVhdGl2ZWNvbW1vbnMub3JnL25zIyIgeG1sbnM6ZGM9Imh0dHA6Ly9wdXJsLm9yZy9kYy9lbGVtZW50cy8xLjEvIiB4bWxuczppbmtzY2FwZT0iaHR0cDovL3d3dy5pbmtzY2FwZS5vcmcvbmFtZXNw ...(+2420 chars)\",\"srcOrientation\":\"Right\"},\"needleOffset\":[-0.8044596912521441,-0.0642123287671233],\"needleSize\":{\"height\":0.4337797619047619,\"width\":0.07668067226890757},\"position\":[0.2829861111111111,0.04398634453781513,0.9196428571428571,0.6088789682539683],\"referencePoint\":\"auto\",\"scaleColors\":[],\"scaleColorsSize\":0.2,\"scaleDirection\":\"LR\",\"showLabels\":1,\"showMinorTicks\":0,\"showSpanLine\":1,\"showTicks\":1,\"tickColor\":[252,252,197],\"tickTransparency\":1,\"valueBarColor\":[0,114,189],\"valueBarOffset\":-0.27,\"valueBarSize\":0.1,\"valueBarTransparency\":1}},{\"name\":\"BackgroundImageComponent\",\"settings\":{\"image\":{\"size\":[380,101],\"src\":\"data:image\\/svg+xml;base64,PHN2ZyB4bWxucz0iaHR0cDovL3d3dy53My5vcmcvMjAwMC9zdmciIHhtbG5zOnhsaW5rPSJodHRwOi8vd3d3LnczLm9yZy8xOTk5L3hsaW5rIiB2aWV3Qm94PSIwIDAgMzgwIDEwMSI+PGRlZnM+PHN0eWxlPi5jbHMtMXtmaWxsOiMwMDJiNDI7fS5jbHMtMntmaWxsOiM0MjcwODI7fS5jbHMtM3tmaWxsOnVybCgjcmFkaWFsLWdyYWRpZW50KTt9LmNscy00e2ZpbGw6I2M4YzhjODtzdHJva2U6IzAwMDt9PC9zdHlsZT48cmFkaWFsR3JhZGllbnQgaWQ9InJhZGlhbC1ncmFkaWVudCIgY3g9IjE5MCIgY3k9IjUwLjUiIHI9IjI2OS4yMSIgZ3JhZGllbnRVbml0cz0idXNlclNwYWNlT25Vc2UiPjxzdG9wIG9mZnNldD0iMC4wMSIgc3RvcC1jb2xvcj0iIzNlNGY1OCIvPjxzdG9wIG9mZnNldD0iMC4wNiIgc3RvcC1jb2xvcj0iIzQ0NTc2MSIvPjxzdG9wIG9mZnNldD0iMC4xNSIgc3RvcC1jb2xvcj0iIzU1NmE3NiIvPjxzdG9wIG9mZnNldD0iMC4yNSIgc3RvcC1jb2xvcj0iIzZkODg5NSIvPjxzdG9wIG9mZnNldD0iMC4zOCIgc3RvcC1jb2xvcj0iIzhmYjJjMyIvPjxzdG9wIG9mZnNldD0iMC41MiIgc3RvcC1jb2xvcj0iI2I2ZTRmYSIvPjxzdG9wIG9mZnNldD0iMSIgc3RvcC1jb2xvcj0iIzE1NDY1NyIvPjwvcmFkaWFsR3JhZGllbnQ+PC9kZWZzPjxnIGlkPSJmcmFtZSI+PGcgaWQ9IkxheWVyXzIiIGRhdGEtbmFtZT0iTGF5ZXIgMiI+PGcgaWQ9IkxheWVyXzEtMiIgZGF0YS1uYW1lPSJMYXllciAxLTIiPjxyZWN0IGlkPSJyZWN0MTAzNiIgY2xhc3M9ImNscy0xIiB4PSIxMSIgeT0iMTEiIHdpZHRoPSIzNTgiIGhlaWdodD0iNzkiLz48cGF0aCBpZD0icGF0aDEwMzgiIGNsYXNzPSJjbHMtMiIgZD0iTTgsOFY5M0gzNzJWOFpNMzY5LDkwSDExVjExSDM2OVoiLz48cGF0aCBpZD0icGF0aDEwNDAiIGNsYXNzPSJjbHMtMyIgZD0iTTAsMFYxMDFIMzgwVjBaTTM3Miw5M0g4VjhIMzcyWiIvPjwvZz48L2c+PC9nPjxnIGlkPSJ0cmFjayI+PHBhdGggaWQ9InJlY3QxNjExIiBjbGFzcz0iY2xzLTQiIGQ9Ik0zMy4zNywyNi41OUgzNDYuNjNjNCwwLDcuMjUsMi42LDcuMjUsNS44MWgwYzAsMy4yMS0zLjI1LDUuODItNy4yNSw1LjgySDMzLjM3Yy00LDAtNy4yNS0yLjYxLTcuMjUtNS44MmgwQzI2LjEyLDI5LjE5LDI5LjM3LDI2LjU5LDMzLjM3LDI2LjU5WiIvPjwvZz48L3N2Zz4=\",\"srcOrientation\":\"horizontal\"},\"position\":[0,0,1,1],\"scaleMode\":\"0\"}},{\"name\":\"ForegroundImageComponent\",\"settings\":{\"image\":{\"size\":[0,0],\"src\":\"default\",\"srcOrientation\":[]},\"isForeground\":1,\"position\":[0,0,1,1],\"scaleMode\":\"0\"}}],\"settings\":{\"BindingType\":\"param\",\"aspectRatio\":3.7777777777777777,\"backgroundColor\":[0,0,0,\"1\"],\"backgroundOffset\":0,\"backgroundOpacity\":1,\"fixedAspectRatio\":\"on\",\"foregroundColor\":[252,252,196],\"orientation\":\"horizontal\",\"showBackgroundColor\":false,\"value\":0,\"version\":\"R2022b\"},\"type\":\"LinearGauge\"}"
  Steering Angle 1 : CustomTuningWebBlock  LabelPosition=Hide  ShowInitialText=on  Configuration="{\"components\":[{\"name\":\"LinearScaleComponent\",\"settings\":{\"bounds\":{\"max\":100,\"min\":0,\"tickInterval\":\"auto\"},\"internalTickHeightScaleFactor\":0.5,\"labelColor\":[255,255,200],\"labelFont\":{\"font\":\"Arial\",\"fontSize\":12},\"labelOffset\":0.05,\"labelTransparency\":1,\"needleImage\":{\"size\":[596,842],\"src\":\"data:image\\/svg+xml;base64,PD94bWwgdmVyc2lvbj0iMS4wIiBlbmNvZGluZz0idXRmLTgiPz4NCjwhLS0gR2VuZXJhdG9yOiBBZG9iZSBJbGx1c3RyYXRvciAyNS4wLjAsIFNWRyBFeHBvcnQgUGx1Zy1JbiAuIFNWRyBWZXJzaW9uOiA2LjAwIEJ1aWxkIDApICAtLT4NCjxzdmcgdmVyc2lvbj0iMS4xIg0KCSBpZD0ic3ZnOCIgeG1sbnM6Y2M9Imh0dHA6Ly9jcmVhdGl2ZWNvbW1vbnMub3JnL25zIyIgeG1sbnM6ZGM9Imh0dHA6Ly9wdXJsLm9yZy9kYy9lbGVtZW50cy8xLjEvIiB4bWxuczppbmtzY2FwZT0iaHR0cDovL3d3dy5pbmtzY2FwZS5vcmcvbmFtZXNw ...(+2420 chars)\",\"srcOrientation\":\"Right\"},\"needleOffset\":[-0.8044596912521441,-0.0642123287671233],\"needleSize\":{\"height\":0.4337797619047619,\"width\":0.07668067226890757},\"position\":[0.2829861111111111,0.04398634453781513,0.9196428571428571,0.6088789682539683],\"referencePoint\":\"auto\",\"scaleColors\":[],\"scaleColorsSize\":0.2,\"scaleDirection\":\"LR\",\"showLabels\":1,\"showMinorTicks\":0,\"showSpanLine\":1,\"showTicks\":1,\"tickColor\":[252,252,197],\"tickTransparency\":1,\"valueBarColor\":[0,114,189],\"valueBarOffset\":-0.27,\"valueBarSize\":0.1,\"valueBarTransparency\":1}},{\"name\":\"BackgroundImageComponent\",\"settings\":{\"image\":{\"size\":[380,101],\"src\":\"data:image\\/svg+xml;base64,PHN2ZyB4bWxucz0iaHR0cDovL3d3dy53My5vcmcvMjAwMC9zdmciIHhtbG5zOnhsaW5rPSJodHRwOi8vd3d3LnczLm9yZy8xOTk5L3hsaW5rIiB2aWV3Qm94PSIwIDAgMzgwIDEwMSI+PGRlZnM+PHN0eWxlPi5jbHMtMXtmaWxsOiMwMDJiNDI7fS5jbHMtMntmaWxsOiM0MjcwODI7fS5jbHMtM3tmaWxsOnVybCgjcmFkaWFsLWdyYWRpZW50KTt9LmNscy00e2ZpbGw6I2M4YzhjODtzdHJva2U6IzAwMDt9PC9zdHlsZT48cmFkaWFsR3JhZGllbnQgaWQ9InJhZGlhbC1ncmFkaWVudCIgY3g9IjE5MCIgY3k9IjUwLjUiIHI9IjI2OS4yMSIgZ3JhZGllbnRVbml0cz0idXNlclNwYWNlT25Vc2UiPjxzdG9wIG9mZnNldD0iMC4wMSIgc3RvcC1jb2xvcj0iIzNlNGY1OCIvPjxzdG9wIG9mZnNldD0iMC4wNiIgc3RvcC1jb2xvcj0iIzQ0NTc2MSIvPjxzdG9wIG9mZnNldD0iMC4xNSIgc3RvcC1jb2xvcj0iIzU1NmE3NiIvPjxzdG9wIG9mZnNldD0iMC4yNSIgc3RvcC1jb2xvcj0iIzZkODg5NSIvPjxzdG9wIG9mZnNldD0iMC4zOCIgc3RvcC1jb2xvcj0iIzhmYjJjMyIvPjxzdG9wIG9mZnNldD0iMC41MiIgc3RvcC1jb2xvcj0iI2I2ZTRmYSIvPjxzdG9wIG9mZnNldD0iMSIgc3RvcC1jb2xvcj0iIzE1NDY1NyIvPjwvcmFkaWFsR3JhZGllbnQ+PC9kZWZzPjxnIGlkPSJmcmFtZSI+PGcgaWQ9IkxheWVyXzIiIGRhdGEtbmFtZT0iTGF5ZXIgMiI+PGcgaWQ9IkxheWVyXzEtMiIgZGF0YS1uYW1lPSJMYXllciAxLTIiPjxyZWN0IGlkPSJyZWN0MTAzNiIgY2xhc3M9ImNscy0xIiB4PSIxMSIgeT0iMTEiIHdpZHRoPSIzNTgiIGhlaWdodD0iNzkiLz48cGF0aCBpZD0icGF0aDEwMzgiIGNsYXNzPSJjbHMtMiIgZD0iTTgsOFY5M0gzNzJWOFpNMzY5LDkwSDExVjExSDM2OVoiLz48cGF0aCBpZD0icGF0aDEwNDAiIGNsYXNzPSJjbHMtMyIgZD0iTTAsMFYxMDFIMzgwVjBaTTM3Miw5M0g4VjhIMzcyWiIvPjwvZz48L2c+PC9nPjxnIGlkPSJ0cmFjayI+PHBhdGggaWQ9InJlY3QxNjExIiBjbGFzcz0iY2xzLTQiIGQ9Ik0zMy4zNywyNi41OUgzNDYuNjNjNCwwLDcuMjUsMi42LDcuMjUsNS44MWgwYzAsMy4yMS0zLjI1LDUuODItNy4yNSw1LjgySDMzLjM3Yy00LDAtNy4yNS0yLjYxLTcuMjUtNS44MmgwQzI2LjEyLDI5LjE5LDI5LjM3LDI2LjU5LDMzLjM3LDI2LjU5WiIvPjwvZz48L3N2Zz4=\",\"srcOrientation\":\"horizontal\"},\"position\":[0,0,1,1],\"scaleMode\":\"0\"}},{\"name\":\"ForegroundImageComponent\",\"settings\":{\"image\":{\"size\":[0,0],\"src\":\"default\",\"srcOrientation\":[]},\"isForeground\":1,\"position\":[0,0,1,1],\"scaleMode\":\"0\"}}],\"settings\":{\"BindingType\":\"param\",\"aspectRatio\":3.7777777777777777,\"backgroundColor\":[0,0,0,\"1\"],\"backgroundOffset\":0,\"backgroundOpacity\":1,\"fixedAspectRatio\":\"on\",\"foregroundColor\":[252,252,196],\"orientation\":\"horizontal\",\"showBackgroundColor\":false,\"value\":0,\"version\":\"R2022b\"},\"type\":\"LinearGauge\"}"
  Vertical Slider{,1..3} (4 alike) : CustomTuningWebBlock  LabelPosition=Hide  ShowInitialText=on  Configuration="{\"components\":[{\"name\":\"LinearScaleComponent\",\"settings\":{\"bounds\":{\"max\":1,\"min\":0,\"tickInterval\":\"auto\"},\"internalTickHeightScaleFactor\":0.5,\"labelColor\":[255,255,200],\"labelFont\":{\"font\":\"Arial\",\"fontSize\":12},\"labelOffset\":0.05,\"labelTransparency\":1,\"needleImage\":{\"size\":[596,842],\"src\":\"data:image\\/svg+xml;base64,PD94bWwgdmVyc2lvbj0iMS4wIiBlbmNvZGluZz0idXRmLTgiPz4NCjwhLS0gR2VuZXJhdG9yOiBBZG9iZSBJbGx1c3RyYXRvciAyNS4wLjAsIFNWRyBFeHBvcnQgUGx1Zy1JbiAuIFNWRyBWZXJzaW9uOiA2LjAwIEJ1aWxkIDApICAtLT4NCjxzdmcgdmVyc2lvbj0iMS4xIg0KCSBpZD0ic3ZnOCIgeG1sbnM6Y2M9Imh0dHA6Ly9jcmVhdGl2ZWNvbW1vbnMub3JnL25zIyIgeG1sbnM6ZGM9Imh0dHA6Ly9wdXJsLm9yZy9kYy9lbGVtZW50cy8xLjEvIiB4bWxuczppbmtzY2FwZT0iaHR0cDovL3d3dy5pbmtzY2FwZS5vcmcvbmFtZXNw ...(+2420 chars)\",\"srcOrientation\":\"horizontal\"},\"needleOffset\":[0.0642123287671233,-0.8044596912521441],\"needleSize\":{\"height\":0.07668067226890757,\"width\":0.4337797619047619},\"position\":[0.03623949579831933,0.2829861111111111,0.6088789682539683,0.9196428571428571],\"referencePoint\":\"auto\",\"scaleColors\":[],\"scaleColorsSize\":0.2,\"scaleDirection\":\"BT\",\"showLabels\":1,\"showMinorTicks\":0,\"showSpanLine\":1,\"showTicks\":1,\"tickColor\":[252,252,197],\"tickTransparency\":1,\"valueBarColor\":[0,114,189],\"valueBarOffset\":-0.27,\"valueBarSize\":0.1,\"valueBarTransparency\":1}},{\"name\":\"BackgroundImageComponent\",\"settings\":{\"image\":{\"size\":[380,101],\"src\":\"data:image\\/svg+xml;base64,PHN2ZyB4bWxucz0iaHR0cDovL3d3dy53My5vcmcvMjAwMC9zdmciIHhtbG5zOnhsaW5rPSJodHRwOi8vd3d3LnczLm9yZy8xOTk5L3hsaW5rIiB2aWV3Qm94PSIwIDAgMzgwIDEwMSI+PGRlZnM+PHN0eWxlPi5jbHMtMXtmaWxsOiMwMDJiNDI7fS5jbHMtMntmaWxsOiM0MjcwODI7fS5jbHMtM3tmaWxsOnVybCgjcmFkaWFsLWdyYWRpZW50KTt9LmNscy00e2ZpbGw6I2M4YzhjODtzdHJva2U6IzAwMDt9PC9zdHlsZT48cmFkaWFsR3JhZGllbnQgaWQ9InJhZGlhbC1ncmFkaWVudCIgY3g9IjE5MCIgY3k9IjUwLjUiIHI9IjI2OS4yMSIgZ3JhZGllbnRVbml0cz0idXNlclNwYWNlT25Vc2UiPjxzdG9wIG9mZnNldD0iMC4wMSIgc3RvcC1jb2xvcj0iIzNlNGY1OCIvPjxzdG9wIG9mZnNldD0iMC4wNiIgc3RvcC1jb2xvcj0iIzQ0NTc2MSIvPjxzdG9wIG9mZnNldD0iMC4xNSIgc3RvcC1jb2xvcj0iIzU1NmE3NiIvPjxzdG9wIG9mZnNldD0iMC4yNSIgc3RvcC1jb2xvcj0iIzZkODg5NSIvPjxzdG9wIG9mZnNldD0iMC4zOCIgc3RvcC1jb2xvcj0iIzhmYjJjMyIvPjxzdG9wIG9mZnNldD0iMC41MiIgc3RvcC1jb2xvcj0iI2I2ZTRmYSIvPjxzdG9wIG9mZnNldD0iMSIgc3RvcC1jb2xvcj0iIzE1NDY1NyIvPjwvcmFkaWFsR3JhZGllbnQ+PC9kZWZzPjxnIGlkPSJmcmFtZSI+PGcgaWQ9IkxheWVyXzIiIGRhdGEtbmFtZT0iTGF5ZXIgMiI+PGcgaWQ9IkxheWVyXzEtMiIgZGF0YS1uYW1lPSJMYXllciAxLTIiPjxyZWN0IGlkPSJyZWN0MTAzNiIgY2xhc3M9ImNscy0xIiB4PSIxMSIgeT0iMTEiIHdpZHRoPSIzNTgiIGhlaWdodD0iNzkiLz48cGF0aCBpZD0icGF0aDEwMzgiIGNsYXNzPSJjbHMtMiIgZD0iTTgsOFY5M0gzNzJWOFpNMzY5LDkwSDExVjExSDM2OVoiLz48cGF0aCBpZD0icGF0aDEwNDAiIGNsYXNzPSJjbHMtMyIgZD0iTTAsMFYxMDFIMzgwVjBaTTM3Miw5M0g4VjhIMzcyWiIvPjwvZz48L2c+PC9nPjxnIGlkPSJ0cmFjayI+PHBhdGggaWQ9InJlY3QxNjExIiBjbGFzcz0iY2xzLTQiIGQ9Ik0zMy4zNywyNi41OUgzNDYuNjNjNCwwLDcuMjUsMi42LDcuMjUsNS44MWgwYzAsMy4yMS0zLjI1LDUuODItNy4yNSw1LjgySDMzLjM3Yy00LDAtNy4yNS0yLjYxLTcuMjUtNS44MmgwQzI2LjEyLDI5LjE5LDI5LjM3LDI2LjU5LDMzLjM3LDI2LjU5WiIvPjwvZz48L3N2Zz4=\",\"srcOrientation\":\"horizontal\"},\"position\":[0,0,1,1],\"scaleMode\":\"0\"}},{\"name\":\"ForegroundImageComponent\",\"settings\":{\"image\":{\"size\":[0,0],\"src\":\"default\",\"srcOrientation\":[]},\"isForeground\":1,\"position\":[0,0,1,1],\"scaleMode\":\"0\"}}],\"settings\":{\"BindingType\":\"param\",\"aspectRatio\":3.7777777777777777,\"backgroundColor\":[0,0,0,\"1\"],\"backgroundOffset\":0,\"backgroundOpacity\":1,\"fixedAspectRatio\":\"on\",\"foregroundColor\":[252,252,196],\"orientation\":\"vertical\",\"showBackgroundColor\":false,\"value\":0,\"version\":\"R2022b\"},\"type\":\"LinearGauge\"}"
